simulink model "MovTraSimulink"  (R2023a)
settings: Solver=VariableStepAuto  StartTime=0.0  StopTime=10.0  MaxStep=time  RelTol=1e-3
values from neighbouring files (symbols this model uses):
  b1 = 1000    [Movsim.m]    (also in ODE45T.m)
  f = 0    [Movsim.m]    (also in ODE45T.m)
  k1 = 16182    [Movsim.m]    (also in ODE45T.m)
  k2 = 19000    [Movsim.m]    (also in ODE45T.m)
  m1 = 290    [Movsim.m]    (also in ODE45T.m)
  m2 = 59    [Movsim.m]    (also in ODE45T.m)
libraries: simulink x2
settings Model: Creator=mluser  LastModifiedBy=eveli
settings OptimizationCC: ReuseModelBlockBuffer=off

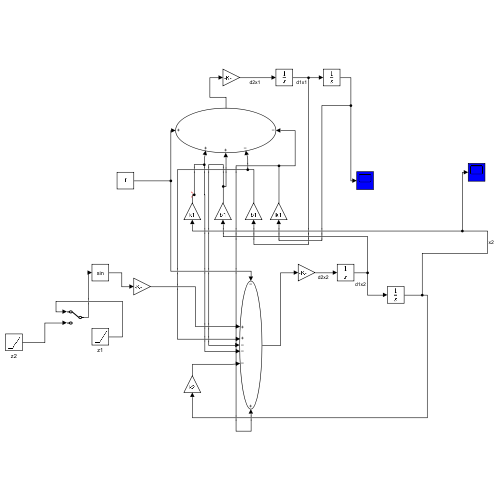
[thumbnail: Simulink's stored preview of the top-level diagram]
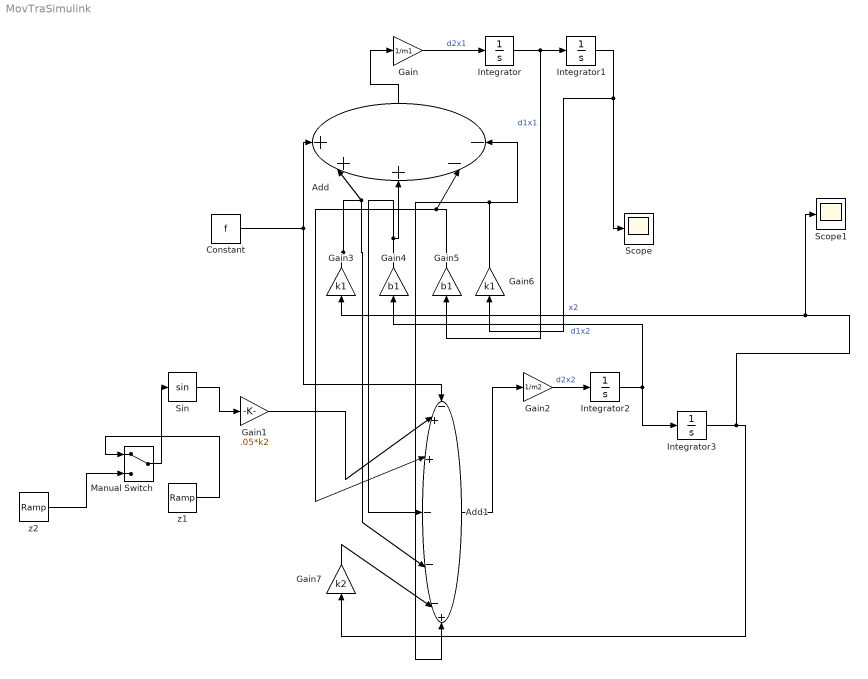
== system MovTraSimulink ==
  Add : Sum  Inputs=+++--
  Add1 : Sum  Inputs=-++---+
  Constant : Constant  Value=f
  Gain : Gain  Gain=1/m1
  Gain1 : Gain  Gain=.05*k2
  Gain2 : Gain  Gain=1/m2
  Gain3 : Gain  Gain=k1
  Gain4 : Gain  Gain=b1
  Gain5 : Gain  Gain=b1
  Gain6 : Gain  Gain=k1
  Gain7 : Gain  Gain=k2
  Integrator{,1..3} (4 alike) : Integrator
  Manual Switch : ManualSwitch
  Scope : Scope
  Scope1 : Scope
  Sin : Trigonometry
  z1 : simulink/Sources/Ramp  slope=.5*pi  start=0  InitialOutput=0
  z2 : simulink/Sources/Ramp  slope=20*pi  start=0  InitialOutput=0
  wires:
  Gain/1 -> Integrator/1  "d2x1"
  Integrator/1 -> Gain5/1, Integrator1/1  "d1x1"
  Add/1 -> Gain/1
  Constant/1 -> Add1/1, Add/1
  Sin/1 -> Gain1/1
  Gain2/1 -> Integrator2/1  "d2x2"
  Integrator2/1 -> Gain4/1, Integrator3/1  "d1x2"
  Gain3/1 -> Add1/5, Add/2
  Integrator3/1 -> Gain7/1, Scope1/1, Gain3/1  "x2"
  Gain4/1 -> Add/3, Add1/4
  Integrator1/1 -> Scope/1, Gain6/1
  Add1/1 -> Gain2/1
  Gain1/1 -> Add1/2
  Gain7/1 -> Add1/6
  z1/1 -> Manual Switch/1
  z2/1 -> Manual Switch/2
  Manual Switch/1 -> Sin/1
  Gain5/1 -> Add1/3, Add/4
  Gain6/1 -> Add1/7, Add/5
